simulink model "W2_counter"  (R2020b)
settings: Solver=VariableStepAuto  StartTime=0.0  StopTime=10.0  RelTol=1e-3
settings Model: Creator=mluser  LastModifiedBy=mluser

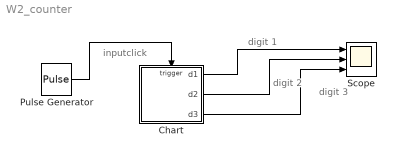
== system W2_counter ==
  note: digit 3
  note: digit 2
  note: digit 1
  note: inputclick
  Chart : Stateflow chart  TreatAsAtomicUnit=on
  Pulse Generator : DiscretePulseGenerator  PulseType=Time based  Period=0.1  PulseWidth=5
  Scope : Scope  NumInputPorts=3
  wires:
  Chart/1(d1) -> Scope/1
  Pulse Generator/1 -> Chart/Trigger
  Chart/3(d3) -> Scope/3
  Chart/2(d2) -> Scope/2

== stateflow chart W2_counter/Chart ==
  state digit1 [parallel]
    settings: executionOrder=1
    state one
      en:d1=1;
    state zero
      en:d1=0;
    state two
      en:d1=2;
    digit1.one -> digit1.two
    digit1.zero -> digit1.one : inputClick
    (default) -> digit1.zero
    digit1.two -> digit1.zero : inputClick/{inc2;}
  state digit2 [parallel]
    settings: executionOrder=2
    state one
      en:d2=1;
    state zero
      en:d2=0;
    state two
      en:d2=2;
    digit2.one -> digit2.two : inc2
    digit2.zero -> digit2.one : inc2
    (default) -> digit2.zero
    digit2.two -> digit2.zero : inc2/{inc3;}
  state digit3 [parallel]
    settings: executionOrder=3
    state one
      en:d3=1;
    state zero
      en:d3=0;
    state two
      en:d3=2;
    digit3.one -> digit3.two : inc3
    digit3.zero -> digit3.one : inc3
    (default) -> digit3.zero
    digit3.two -> digit3.zero : inc3
  data: d1 output; d2 output; d3 output
  events: inputClick input RISING_EDGE_EVENT; inc2 local FUNCTION_CALL_EVENT; inc3 local FUNCTION_CALL_EVENT
